simulink model "closed_loop"  (R2019a)
settings: Solver=FixedStepAuto  StartTime=0.0  StopTime=10  FixedStep=1/100  RelTol=1e-3  AbsTol=1e-3
model workspace: external: MATLAB File params.m (data not in the file)
undefined symbols (not defined in the file or in its folder): g, m, Ts
libraries: nesl_utility x9
settings Model: Creator=Jocke  LastModifiedBy=parke
settings SolverCC: AutoScaleAbsTol=off
settings DataIOCC: ReturnWorkspaceOutputs=off
settings OptimizationCC: UseDivisionForNetSlopeComputation=on
settings DebuggingCC: ArithmeticOperatorsInVariantConditions=warning
settings SFSimCC: SimUseLocalCustomCode=off
settings RTWCC: RTWUseLocalCustomCode=off  Toolchain=GNU gcc/g++ | gmake (64-bit Linux)
settings CodeAppCC: StateflowObjectComments=on
settings SimscapeCC: SimscapeNormalizeSystem=off  SimscapeLogType=all  SimscapeLogDataHistory=10000

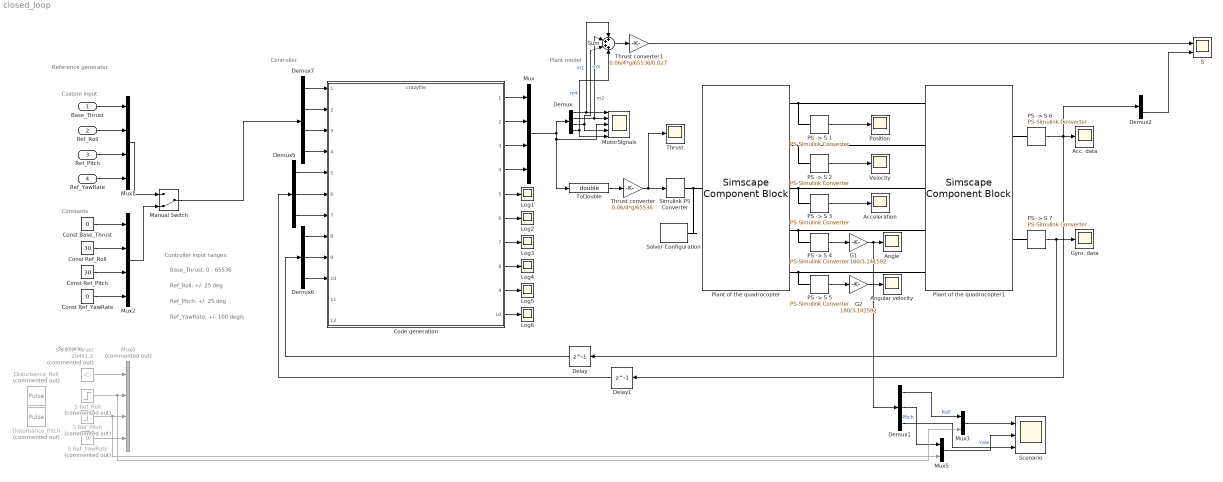
== system closed_loop ==
  note: Custom input
  note: Plant model
  note: Controller
  note: Constants
  note: Reference generator
  note: Ref_Roll: +/- 25 deg
  note: Base_Thrust: 0 - 65536
  note: Ref_Pitch: +/- 25 deg
  note: Ref_YawRate: +/- 100 deg/s
  note: Controller input ranges:
  note: Scenario
  Base_Thrust : Inport  OutDataTypeStr=double
  Ref_Roll : Inport  Port=2  OutDataTypeStr=double
  Ref_Pitch : Inport  Port=3  OutDataTypeStr=double
  Ref_YawRate : Inport  Port=4  OutDataTypeStr=double
  Acc. data : Scope
  Acceleration : Scope
  Angle : Scope
  Angular velocity : Scope
  Code generation : ModelReference  ModelNameDialog=crazyflie.slx  SimulationMode=Normal  ModelReferenceVersion=1.224
  Const Base_Thrust : Constant  Value=0  SampleTime=Ts
  Const Ref_Pitch : Constant  Value=30
  Const Ref_Roll : Constant  Value=30
  Const Ref_YawRate : Constant  Value=0
  Delay : Delay  DelayLength=1
  Delay1 : Delay  DelayLength=1
  Demux : Demux
  Demux{1..2,5..6} (4 alike) : Demux  Outputs=3
  Demux7 : Demux
  Disturbance_Pitch : DiscretePulseGenerator  Commented=on  PulseType=Time based  Amplitude=6  Period=10  PhaseDelay=6
  Disturbance_Roll : DiscretePulseGenerator  Commented=on  PulseType=Time based  Amplitude=6  Period=10  PhaseDelay=4
  G1 : Gain  Gain=180/3.141592
  G2 : Gain  Gain=180/3.141592
  Gyro. data : Scope
  Log{1..6} (6 alike) : Scope
  Manual Switch : ManualSwitch  CurrentSetting=0
  MotorSignals : Scope  NumInputPorts=5
  Mux : Mux
  Mux1 : Mux
  Mux2 : Mux
  Mux3 : Mux  Inputs=2
  Mux4 : Mux  Commented=on
  Mux5 : Mux  Inputs=2
  PS -> S {1..7} (7 alike) : nesl_utility/PS-Simulink Converter  PhysicalDomain=network_engine_domain  SubClassName=ps_output  LeftPortType=input  RightPortType=output  PseudoPeriodic=off  Frequencies=[]  Unit=1  AffineConversion=off
  Plant of the quadrocopter : SimscapeComponentBlock  SourceFile=plant  ComponentPath=plant  ComponentVariants=plant  ComponentVariantNames=plant  ClassName=plant  SchemaVersion=1  m=m kg  g=g m/s^2  d=d m  k=2.5383e-11 m  b=1.9796e-9
      settings: CopyFcn=simscape.engine.sli.internal.componentblockcallback(gcbh,'COPY')  PreCopyFcn=simscape.engine.sli.internal.componentblockcallback(gcbh,'PRECOPY')  PreDeleteFcn=simscape.engine.sli.internal.componentblockcallback(gcbh,'PREDELETE')
      mask Type: Plant of quadrocopter
  Plant of the quadrocopter1 : SimscapeComponentBlock  SourceFile=sensors_new  ComponentPath=sensors_new  ComponentVariants=sensors_new  ComponentVariantNames=sensors_new  ClassName=sensors_new  SchemaVersion=1
      settings: CopyFcn=simscape.engine.sli.internal.componentblockcallback(gcbh,'COPY')  PreCopyFcn=simscape.engine.sli.internal.componentblockcallback(gcbh,'PRECOPY')  PreDeleteFcn=simscape.engine.sli.internal.componentblockcallback(gcbh,'PREDELETE')
      mask Type: Plant of quadrocopter
  Position : Scope
  S : Scope  NumInputPorts=2
  S Base_Thrust : Constant  Commented=on  Value=29491.2  SampleTime=Ts
  S Ref_Pitch : Step  Commented=on  Time=4  After=10  SampleTime=0
  S Ref_Roll : Step  Commented=on  Time=6  Before=10  After=0  SampleTime=0
  S Ref_YawRate : Constant  Commented=on  Value=0
  Scenario : Scope  NumInputPorts=3
  Simulink-PS Converter : nesl_utility/Simulink-PS Converter  PhysicalDomain=network_engine_domain  SubClassName=ps_input  LeftPortType=input  RightPortType=output  PseudoPeriodic=off  Frequencies=[]  NoiseDistribution=none  NoiseParameters=[]  Unit=1  AffineConversion=off  FilteringAndDerivatives=zero  SimscapeFilterOrder=1  InputFilterTimeConstant=0.001  UdotUserProvided=1
  Solver Configuration : nesl_utility/Solver Configuration  PhysicalDomain=network_engine_domain  SubClassName=solver  LeftPortType=input  RightPortType=generic  Tones=[]  Harmonics=[]  SimulateNoise=off  Profile=off  UseLocalSampling=off  EnableSwitchedLinearOptims=on  FrequencyDomain=off  UseCCode=off  RelTol=0.001  AbsTol=1e-06  MinStep=1e-09  ToWorkspace=off  RevertToSquareIcSolve=off  NumHomotopyIterations=100  PhasorMode=off  PhasorModeNumHarmonics=1  DoDC=off  ResidualTolerance=1e-09  UseLocalSolver=off  LocalSolverChoice=NE_BACKWARD_EULER_ADVANCER  LocalSolverSampleTime=0.001  DoFixedCost=off  MaxNonlinIter=3  MaxModeIter=2  LinearAlgebra=Sparse  EquationFormulation=NE_TIME_EF  DelaysMemoryBudget=1024  AutomaticFiltering=on  FilteringTimeConstant=0.001  PartitionStorageMethod=AS_NEEDED  PartitionMemoryBudget=1024  PartitionMethod=FAST
  Sum : Sum  Inputs=++++
  Thrust : Scope
  Thrust converter : Gain  Gain=0.06/4*g/65536
  Thrust converter1 : Gain  Gain=0.06/4*g/65536/0.027
  ToDouble : DataTypeConversion  OutDataTypeStr=double  RndMeth=Round  SaturateOnIntegerOverflow=on
  Velocity : Scope
  wires:
  Code generation/1 -> Mux/1
  Code generation/4 -> Mux/4
  Code generation/3 -> Mux/3
  Code generation/2 -> Mux/2
  Demux5/1 -> Code generation/5
  Demux5/2 -> Code generation/6
  Demux5/3 -> Code generation/7
  Demux6/1 -> Code generation/8
  Demux6/2 -> Code generation/9
  Demux6/3 -> Code generation/10
  "PS -> S 7"/1 -> Delay/1, Gyro. data/1
  "PS -> S 6"/1 -> Demux2/1, Delay1/1, Acc. data/1
  Code generation/5 -> Log1/1
  Code generation/6 -> Log2/1
  Code generation/7 -> Log3/1
  Code generation/8 -> Log4/1
  Code generation/9 -> Log5/1
  Code generation/10 -> Log6/1
  Mux/1 -> Demux/1, MotorSignals/3, ToDouble/1
  Base_Thrust/1 -> Mux1/1
  Ref_Roll/1 -> Mux1/2
  Ref_Pitch/1 -> Mux1/3
  Ref_YawRate/1 -> Mux1/4
  Mux1/1 -> Manual Switch/1
  Const Base_Thrust/1 -> Mux2/1
  Const Ref_Pitch/1 -> Mux2/3
  Const Ref_YawRate/1 -> Mux2/4
  Manual Switch/1 -> Demux7/1
  Demux7/1 -> Code generation/1
  Demux7/2 -> Code generation/2
  Demux7/3 -> Code generation/3
  Demux7/4 -> Code generation/4
  G1/1 -> Demux1/1, Angle/1
  G2/1 -> Angular velocity/1
  ToDouble/1 -> Thrust converter/1
  Thrust converter/1 -> Thrust/1, Simulink-PS Converter/1
  "PS -> S 1"/1 -> Position/1
  "PS -> S 5"/1 -> G2/1
  "PS -> S 4"/1 -> G1/1
  "PS -> S 3"/1 -> Acceleration/1
  "PS -> S 2"/1 -> Velocity/1
  Delay/1 -> Demux6/1
  Delay1/1 -> Demux5/1
  Demux/1 -> Sum/1, MotorSignals/1  "m1"
  Demux/2 -> Sum/2, MotorSignals/2  "m2"
  Demux/3 -> Sum/3, MotorSignals/4  "m3"
  Demux/4 -> Sum/4, MotorSignals/5  "m4"
  S Base_Thrust/1 -> Mux4/1
  S Ref_YawRate/1 -> Mux4/4
  Mux3/1 -> Scenario/1
  Mux5/1 -> Scenario/2
  Demux1/1 -> Mux3/1  "Roll"
  Demux1/2 -> Mux5/1  "Pitch"
  Demux1/3 -> Scenario/3  "Yaw"
  Mux2/1 -> Manual Switch/2
  Sum/1 -> Thrust converter1/1
  Thrust converter1/1 -> S/1
  Demux2/3 -> S/2
  Const Ref_Roll/1 -> Mux2/2
  S Ref_Roll/1 -> Mux4/2, Mux3/2
  S Ref_Pitch/1 -> Mux5/2, Mux4/3
  connections:
  Simulink-PS Converter/RConn1 -- Solver Configuration/RConn1 -- Plant of the quadrocopter/LConn1
  Plant of the quadrocopter1/LConn1 -- "PS -> S 1"/LConn1 -- Plant of the quadrocopter/RConn1
  Plant of the quadrocopter1/LConn2 -- "PS -> S 2"/LConn1 -- Plant of the quadrocopter/RConn2
  Plant of the quadrocopter1/LConn3 -- "PS -> S 3"/LConn1 -- Plant of the quadrocopter/RConn3
  Plant of the quadrocopter1/LConn4 -- "PS -> S 4"/LConn1 -- Plant of the quadrocopter/RConn4
  Plant of the quadrocopter1/LConn5 -- "PS -> S 5"/LConn1 -- Plant of the quadrocopter/RConn5
  Plant of the quadrocopter1/RConn1 -- "PS -> S 6"/LConn1
  Plant of the quadrocopter1/RConn2 -- "PS -> S 7"/LConn1
